simulink model "Azimut3"  (R2025b)
settings: Solver=VariableStepAuto  StartTime=0.0  StopTime=30.0  RelTol=1e-3
libraries: simulink x1
settings Model: Creator=alfon  LastModifiedBy=alfon

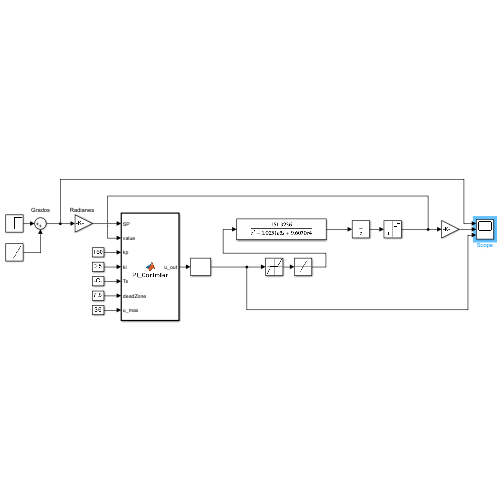
[thumbnail: Simulink's stored preview of the top-level diagram]
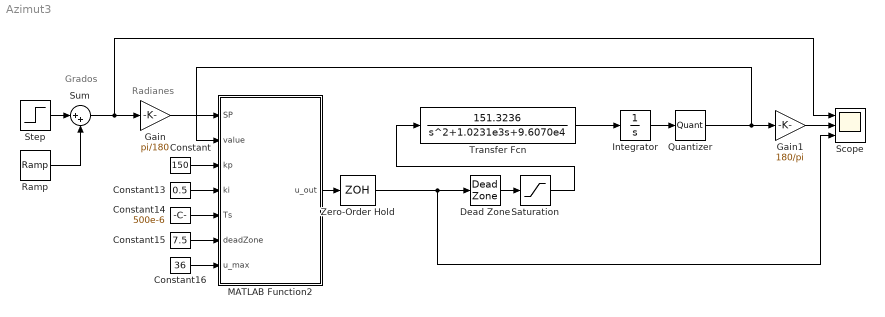
== system Azimut3 ==
  note: Grados
  note: Radianes
  Constant : Constant  Value=150
  Constant13 : Constant  Value=0.5
  Constant14 : Constant  Value=500e-6
  Constant15 : Constant  Value=7.5
  Constant16 : Constant  Value=36
  Dead Zone : DeadZone  LowerValue=-7.5  UpperValue=7.5
  Gain : Gain  Gain=pi/180
  Gain1 : Gain  Gain=180/pi
  Integrator : Integrator
  MATLAB Function2 : MATLAB Function  TreatAsAtomicUnit=on  SystemSampleTime=500e-6
  Quantizer : Quantizer  QuantizationInterval=0.2*pi/180
  Ramp : simulink/Sources/Ramp  slope=0.05  start=0  InitialOutput=0
  Saturation : Saturate  UpperLimit=36  LowerLimit=-36
  Scope : Scope  NumInputPorts=3
      settings: ActiveDisplayYMinimum=-4.4999999999999991  ActiveDisplayYMaximum=40.5
  Step : Step  Time=0  After=20  SampleTime=0
  Sum : Sum  Inputs=|++
  Transfer Fcn : TransferFcn  Numerator=[151.3236]  Denominator=[1 1.0231e3 9.6070e4]
  Zero-Order Hold : ZeroOrderHold  SampleTime=-1
  wires:
  Sum/1 -> Scope/1, Gain/1
  Gain1/1 -> Scope/2
  Step/1 -> Sum/1
  Dead Zone/1 -> Saturation/1
  Ramp/1 -> Sum/2
  Integrator/1 -> Quantizer/1
  Saturation/1 -> Transfer Fcn/1
  Quantizer/1 -> Gain1/1, MATLAB Function2/2(value)
  Constant15/1 -> MATLAB Function2/6(deadZone)
  Constant/1 -> MATLAB Function2/3(kp)
  Constant16/1 -> MATLAB Function2/7(u_max)
  Constant13/1 -> MATLAB Function2/4(ki)
  Constant14/1 -> MATLAB Function2/5(Ts)
  Gain/1 -> MATLAB Function2/1(SP)
  MATLAB Function2/1(u_out) -> Zero-Order Hold/1
  Transfer Fcn/1 -> Integrator/1
  Zero-Order Hold/1 -> Scope/3, Dead Zone/1

== matlab function Azimut3/MATLAB Function2 ==
  data: SP input; u_out output; value input; kp input; ki input; Ts input; deadZone input; u_max input
function u_out = PI_Controller(SP, value, kp, ki, Ts, deadZone, u_max)

    persistent e1 u1 v_f

    if isempty(e1)
        e1 = 0;
        u1 = 0;
        v_f = 0;
    end

    % -------- Low-pass filter --------
    fc = 0.5;                           % Hz
    alpha = exp(-2*pi*fc*Ts);
    v_f = alpha*v_f + (1-alpha)*value;

    % -------- PI (Tustin incremental) --------
    a = kp + (ki*Ts)/2;
    b = -kp + (ki*Ts)/2;

    e0 = SP - v_f;
    u0 = u1 + a*e0 + b*e1;

    % -------- Dead-zone compensation --------
    if u0 > 0
        u_dz = u0 + deadZone;
    elseif u0 < 0
        u_dz = u0 - deadZone;
    else
        u_dz = 0;
    end
    
    
    % -------- Saturation --------
    u_sat = min(max(u_dz, -u_max), u_max);

    % -------- Anti-windup --------
    if abs(u_sat) <= u_max
        u1 = u0;
        e1 = e0;
    end

    u_out = u_sat;
end
